simulink model "TVC6DOF_sim"  (R2020b)
settings: Solver=VariableStepAuto  StartTime=0.0  StopTime=7  RelTol=1e-3
values from neighbouring files (symbols this model uses):
  dt = 0.01    [TVC6DOF.m]
  g = 9.81    [TVC6DOF.m]
  Ix_mc = Ix_n+randn*Ix_v    [TVC6DOF.m]
  Ix_n = 0.1    [TVC6DOF.m]
  Iy_mc = Iy_n+randn*Iy_v    [TVC6DOF.m]
  Iy_n = 0.1    [TVC6DOF.m]
  Iz_mc = Iz_n+randn*Iz_v    [TVC6DOF.m]
  Iz_n = 0.1    [TVC6DOF.m]
  kd = 0.1    [TVC6DOF.m]
  ki = 1    [TVC6DOF.m]
  kp = 1    [TVC6DOF.m]
  l_mc = l_n+randn*l_v    [TVC6DOF.m]
  l_n = 0.3    [TVC6DOF.m]
  m_dry_mc = m_dry_n+randn*m_dry_v    [TVC6DOF.m]
  m_dry_n = 0.94    [TVC6DOF.m]
  mis_y_mc = randn*mis_y_v    [TVC6DOF.m]
  mis_z_mc = randn*mis_z_v    [TVC6DOF.m]
  servo_delay_mc = servo_delay_n+randn*servo_delay_v    [TVC6DOF.m]
  static_error_y_mc = randn*static_error_y_v    [TVC6DOF.m]
  static_error_z_mc = randn*static_error_z_v    [TVC6DOF.m]
undefined symbols (not defined in the file or in its folder): sigbuilder_block
settings Model: Creator=govindchari  LastModifiedBy=govindchari

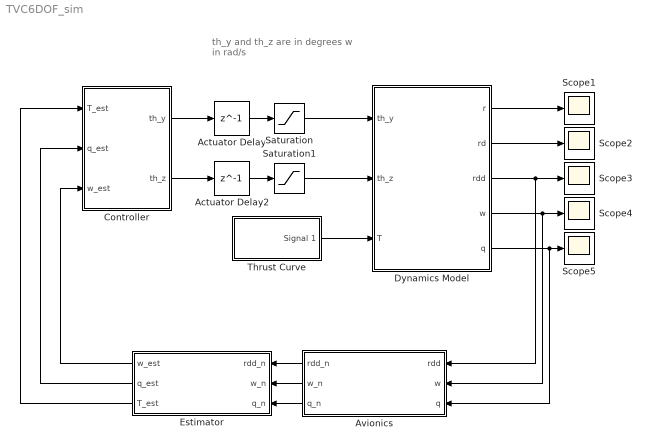
== system TVC6DOF_sim ==
  note: th_y and th_z are in degrees
      |              w in rad/s
  Actuator Delay : Delay  DelayLength=1  InitialCondition=0  SampleTime=servo_delay_mc
  Actuator Delay2 : Delay  DelayLength=1  InitialCondition=0  SampleTime=servo_delay_mc
  Avionics : Subsystem
  Controller : Subsystem
  Dynamics Model : Subsystem
  Estimator : Subsystem
  Saturation : Saturate  UpperLimit=10  LowerLimit=-10
  Saturation1 : Saturate  UpperLimit=10  LowerLimit=-10
  Scope{1..5} (5 alike) : Scope
  Thrust Curve : Subsystem  Tag=STV Subsys  LoadFcn=sigbuilder_block('load');  StartFcn=sigbuilder_block('start');  StopFcn=sigbuilder_block('stop');  ClipboardFcn=sigbuilder_block('clipboard');  mask(Sigbuilder block){tuvar=[0:10]}
      mask help: Simulink:masks:SigbuilderBlock_MD
      mask init:
      | if ~strcmp(get_param(bdroot(gcbh),'SimulationStatus'),'stopped') tuvar = sigbuilder_block('maskInit'); end
      settings: CopyFcn=sigbuilder_block('copy');  DeleteFcn=sigbuilder_block('delete');  ModelCloseFcn=sigbuilder_block('modelClose');  PreSaveFcn=sigbuilder_block('preSave');  PauseFcn=sigbuilder_block('pause');  ContinueFcn=sigbuilder_block('continue');  NameChangeFcn=sigbuilder_block('namechange');  OpenFcn=sigbuilder_block('open',[767 231 550 400 ]);  CloseFcn=sigbuilder_block('close');
      mask Display: plot(0, 0, 100, 100,[2, 2, 32, 32, 2], [68, 8, 8, 68, 68],[32, 2], [38, 38], [32, 19, 2],[53, 60, 44], [32, 17, 17, 2],[16, 16, 31, 31]);txt = getActiveGroup(gcbh);text(2, 100, txt,'verticalAlignment', 'top');
  wires:
  Thrust Curve/1(Signal 1) -> Dynamics Model/3(T)
  Dynamics Model/1(r) -> Scope1/1
  Dynamics Model/2(rd) -> Scope2/1
  Dynamics Model/5(q) -> Avionics/3(q), Scope5/1
  Dynamics Model/4(w) -> Scope4/1, Avionics/2(w)
  Dynamics Model/3(rdd) -> Avionics/1(rdd), Scope3/1
  Avionics/1(rdd_n) -> Estimator/1(rdd_n)
  Avionics/2(w_n) -> Estimator/2(w_n)
  Avionics/3(q_n) -> Estimator/3(q_n)
  Estimator/2(q_est) -> Controller/2(q_est)
  Estimator/3(T_est) -> Controller/1(T_est)
  Controller/2(th_z) -> Actuator Delay2/1
  Actuator Delay2/1 -> Saturation1/1
  Controller/1(th_y) -> Actuator Delay/1
  Actuator Delay/1 -> Saturation/1
  Estimator/1(w_est) -> Controller/3(w_est)
  Saturation/1 -> Dynamics Model/1(th_y)
  Saturation1/1 -> Dynamics Model/2(th_z)

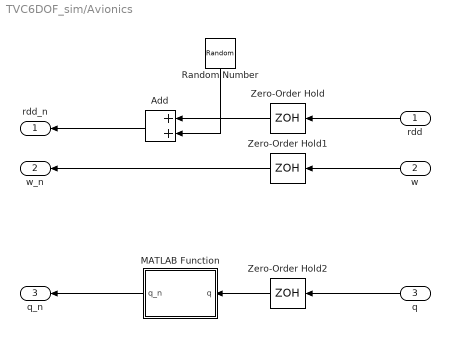
== system TVC6DOF_sim/Avionics ==
  rdd : Inport
  w : Inport  Port=2
  q : Inport  Port=3
  Add : Sum
  MATLAB Function : MATLAB Function  TreatAsAtomicUnit=on
  Random Number : RandomNumber  Mean=0.01  SampleTime=dt
  Zero-Order Hold : ZeroOrderHold  SampleTime=dt
  Zero-Order Hold1 : ZeroOrderHold  SampleTime=dt
  Zero-Order Hold2 : ZeroOrderHold  SampleTime=dt
  rdd_n : Outport
  w_n : Outport  Port=2
  q_n : Outport  Port=3
  wires:
  q/1 -> Zero-Order Hold2/1
  Zero-Order Hold2/1 -> MATLAB Function/1(q)
  w/1 -> Zero-Order Hold1/1
  rdd/1 -> Zero-Order Hold/1
  Zero-Order Hold1/1 -> w_n/1
  Zero-Order Hold/1 -> Add/1
  Add/1 -> rdd_n/1
  Random Number/1 -> Add/2
  MATLAB Function/1(q_n) -> q_n/1

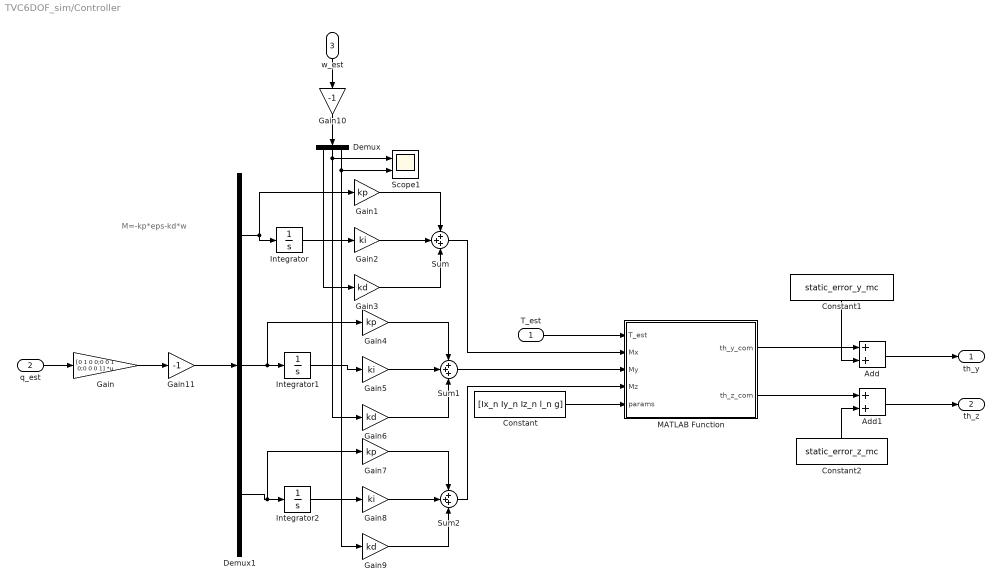
== system TVC6DOF_sim/Controller ==
  note: M=-kp*eps-kd*w
  T_est : Inport
  q_est : Inport  Port=2
  w_est : Inport  Port=3
  Add : Sum
  Add1 : Sum
  Constant : Constant  Value=[Ix_n Iy_n Iz_n l_n g]
  Constant1 : Constant  Value=static_error_y_mc
  Constant2 : Constant  Value=static_error_z_mc
  Demux : Demux  Outputs=3
  Demux1 : Demux  Outputs=3
  Gain : Gain  Gain=[0 1 0 0;0 0 1 0;0 0 0 1]  Multiplication=Matrix(K*u) (u vector)
  Gain1 : Gain  Gain=kp
  Gain10 : Gain  Gain=-1
  Gain11 : Gain  Gain=-1
  Gain2 : Gain  Gain=ki
  Gain3 : Gain  Gain=kd
  Gain4 : Gain  Gain=kp
  Gain5 : Gain  Gain=ki
  Gain6 : Gain  Gain=kd
  Gain7 : Gain  Gain=kp
  Gain8 : Gain  Gain=ki
  Gain9 : Gain  Gain=kd
  Integrator : Integrator  InitialCondition=[0]
  Integrator1 : Integrator  InitialCondition=[0]
  Integrator2 : Integrator  InitialCondition=[0]
  MATLAB Function : MATLAB Function  TreatAsAtomicUnit=on
  Scope1 : Scope  NumInputPorts=2
  Sum : Sum  Inputs=3
  Sum1 : Sum  Inputs=3
  Sum2 : Sum  Inputs=3
  th_y : Outport
  th_z : Outport  Port=2
  wires:
  Integrator/1 -> Gain2/1
  Gain1/1 -> Sum/1
  Gain2/1 -> Sum/2
  Gain3/1 -> Sum/3
  Sum2/1 -> MATLAB Function/4(Mz)
  Sum1/1 -> MATLAB Function/3(My)
  Sum/1 -> MATLAB Function/2(Mx)
  Constant/1 -> MATLAB Function/5(params)
  T_est/1 -> MATLAB Function/1(T_est)
  Demux1/1 -> Integrator/1, Gain1/1
  Integrator1/1 -> Gain5/1
  Gain4/1 -> Sum1/1
  Gain6/1 -> Sum1/3
  Gain5/1 -> Sum1/2
  Demux1/2 -> Gain4/1, Integrator1/1
  Integrator2/1 -> Gain8/1
  Gain7/1 -> Sum2/1
  Gain9/1 -> Sum2/3
  Gain8/1 -> Sum2/2
  Demux1/3 -> Gain7/1, Integrator2/1
  Demux/2 -> Gain6/1, Scope1/1
  Demux/1 -> Gain3/1
  w_est/1 -> Gain10/1
  Gain10/1 -> Demux/1
  q_est/1 -> Gain/1
  Gain/1 -> Gain11/1
  Gain11/1 -> Demux1/1
  Demux/3 -> Scope1/2, Gain9/1
  MATLAB Function/1(th_y_com) -> Add/1
  Add/1 -> th_y/1
  MATLAB Function/2(th_z_com) -> Add1/1
  Add1/1 -> th_z/1
  Constant1/1 -> Add/2
  Constant2/1 -> Add1/2

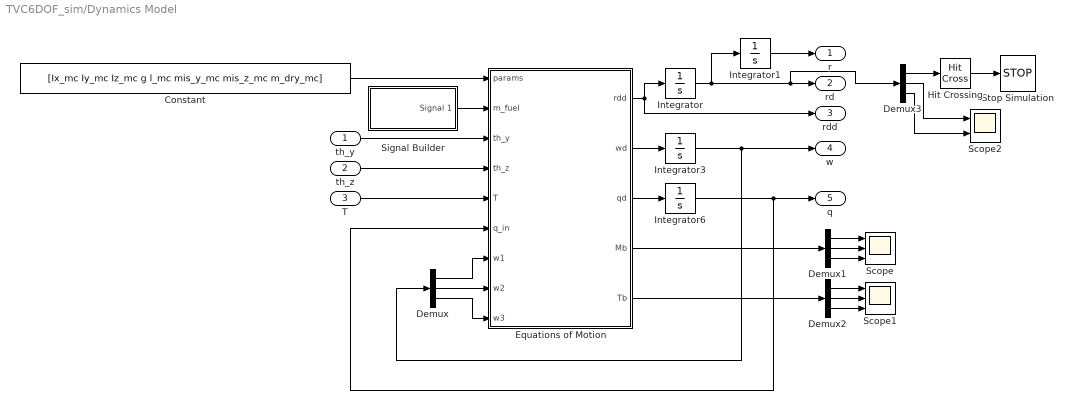
== system TVC6DOF_sim/Dynamics Model ==
  th_y : Inport
  th_z : Inport  Port=2
  T : Inport  Port=3
  Constant : Constant  Value=[Ix_mc Iy_mc Iz_mc g l_mc mis_y_mc mis_z_mc m_dry_mc]
  Demux{,1..3} (4 alike) : Demux  Outputs=3
  Equations of Motion : MATLAB Function  TreatAsAtomicUnit=on
  Hit Crossing : HitCross  HitCrossingOffset=0.01  HitCrossingDirection=falling
  Integrator : Integrator  InitialCondition=[0 0 0]
  Integrator1 : Integrator  InitialCondition=[0 0 0]
  Integrator3 : Integrator  InitialCondition=[0 0 0]
  Integrator6 : Integrator  InitialCondition=[1 0 0 0]
  Scope : Scope  NumInputPorts=3
  Scope1 : Scope  NumInputPorts=3
  Scope2 : Scope  NumInputPorts=2
  Signal Builder : Subsystem  Tag=STV Subsys  LoadFcn=sigbuilder_block('load');  StartFcn=sigbuilder_block('start');  StopFcn=sigbuilder_block('stop');  ClipboardFcn=sigbuilder_block('clipboard');  mask(Sigbuilder block){tuvar=[0:10]}
      mask help: Simulink:masks:SigbuilderBlock_MD
      mask init:
      | if ~strcmp(get_param(bdroot(gcbh),'SimulationStatus'),'stopped') tuvar = sigbuilder_block('maskInit'); end
      settings: CopyFcn=sigbuilder_block('copy');  DeleteFcn=sigbuilder_block('delete');  ModelCloseFcn=sigbuilder_block('modelClose');  PreSaveFcn=sigbuilder_block('preSave');  PauseFcn=sigbuilder_block('pause');  ContinueFcn=sigbuilder_block('continue');  NameChangeFcn=sigbuilder_block('namechange');  OpenFcn=sigbuilder_block('open',[226 376 550 400 ]);  CloseFcn=sigbuilder_block('close');
      mask Display: plot(0, 0, 100, 100,[2, 2, 32, 32, 2], [68, 8, 8, 68, 68],[32, 2], [38, 38], [32, 19, 2],[53, 60, 44], [32, 17, 17, 2],[16, 16, 31, 31]);txt = getActiveGroup(gcbh);text(2, 100, txt,'verticalAlignment', 'top');
  Stop Simulation : Stop
  r : Outport
  rd : Outport  Port=2
  rdd : Outport  Port=3
  w : Outport  Port=4
  q : Outport  Port=5
  wires:
  Constant/1 -> Equations of Motion/1(params)
  th_y/1 -> Equations of Motion/3(th_y)
  th_z/1 -> Equations of Motion/4(th_z)
  Equations of Motion/3(qd) -> Integrator6/1
  Equations of Motion/2(wd) -> Integrator3/1
  Equations of Motion/1(rdd) -> Integrator/1, rdd/1
  T/1 -> Equations of Motion/5(T)
  Integrator/1 -> Integrator1/1, Demux3/1, rd/1
  Integrator1/1 -> r/1
  Demux/1 -> Equations of Motion/7(w1)
  Demux/2 -> Equations of Motion/8(w2)
  Demux/3 -> Equations of Motion/9(w3)
  Integrator6/1 -> Equations of Motion/6(q_in), q/1
  Integrator3/1 -> Demux/1, w/1
  Equations of Motion/4(Mb) -> Demux1/1
  Equations of Motion/5(Tb) -> Demux2/1
  Demux1/1 -> Scope/1
  Demux1/2 -> Scope/2
  Demux1/3 -> Scope/3
  Demux2/1 -> Scope1/1
  Demux2/2 -> Scope1/2
  Demux2/3 -> Scope1/3
  Signal Builder/1(Signal 1) -> Equations of Motion/2(m_fuel)
  Demux3/1 -> Hit Crossing/1
  Hit Crossing/1 -> Stop Simulation/1
  Demux3/2 -> Scope2/1
  Demux3/3 -> Scope2/2

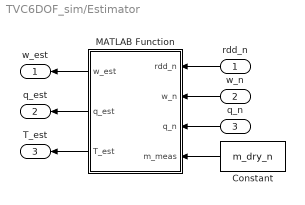
== system TVC6DOF_sim/Estimator ==
  rdd_n : Inport
  w_n : Inport  Port=2
  q_n : Inport  Port=3
  Constant : Constant  Value=m_dry_n
  MATLAB Function : MATLAB Function  TreatAsAtomicUnit=on
  w_est : Outport
  q_est : Outport  Port=2
  T_est : Outport  Port=3
  wires:
  w_n/1 -> MATLAB Function/2(w_n)
  rdd_n/1 -> MATLAB Function/1(rdd_n)
  q_n/1 -> MATLAB Function/3(q_n)
  Constant/1 -> MATLAB Function/4(m_meas)
  MATLAB Function/2(q_est) -> q_est/1
  MATLAB Function/3(T_est) -> T_est/1
  MATLAB Function/1(w_est) -> w_est/1

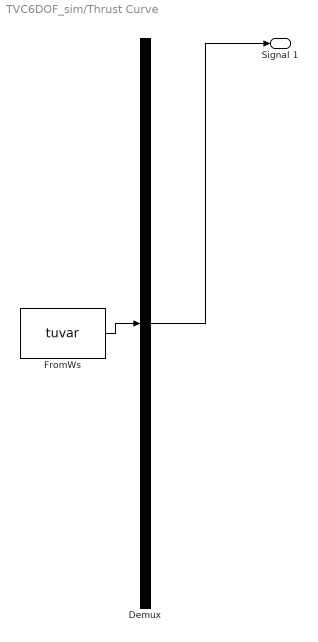
== system TVC6DOF_sim/Thrust Curve ==
  Demux : Demux  Tag=STV Demux  Outputs=1
      settings: DisplayOption=none
  FromWs : FromWorkspace  Tag=STV FromWs  VariableName=tuvar
      SigBuilderData=|
      | common.afterFinalStr = 'Extrapolate'
      | common.sampleTime = 0
      | dataSet.timeRange = [0 10]
      | dataSet.name = 'Group 1'
      | sbobj.Groups.Name = 'Group 1'
      | sbobj.Groups.Signals.Name = 'Signal 1'
      | sbobj.Groups.Signals.XData = [0 0.148 0.228 0.294 0.353 0.382 0.419 0.477 0.52 0.593 0.688 0.855 1.037 1.205 1.423 1.452 1.503 1.736 1.955 2.21 2.494 2.763 3.12 3.382 3.404 3.418 3.45 10]
      | sbobj.Groups.Signals.YData = [0 7.638 12.253 16.391 20.21 22.756 25.26 23.074 20.845 19.093 17.5 16.225 15.427 14.948 14.627 15.741 14.785 14.623 14.303 14.141 13.819 13.338 13.334 13.013 9.352 4.895 0 0]
  Signal 1 : Outport  Tag=STV Outport
  wires:
  Demux/1 -> Signal 1/1
  FromWs/1 -> Demux/1

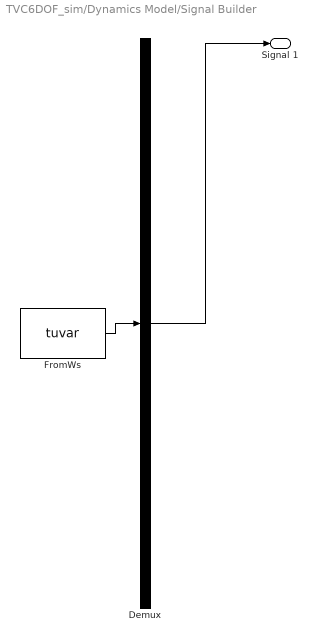
== system TVC6DOF_sim/Dynamics Model/Signal Builder ==
  Demux : Demux  Tag=STV Demux  Outputs=1
      settings: DisplayOption=none
  FromWs : FromWorkspace  Tag=STV FromWs  VariableName=tuvar
      SigBuilderData=|
      | common.afterFinalStr = 'Extrapolate'
      | common.sampleTime = 0
      | dataSet.timeRange = [0 10]
      | dataSet.name = 'Group 1'
      | sbobj.Groups.Name = 'Group 1'
      | sbobj.Groups.Signals.Name = 'Signal 1'
      | sbobj.Groups.Signals.XData = [0 0.148 0.228 0.294 0.419 0.477 0.52 0.593 0.688 0.855 1.037 1.205 1.423 1.452 1.503 1.736 1.955 2.21 2.494 2.763 3.12 3.382 3.404 3.418 3.45 9.8 10]
      | sbobj.Groups.Signals.YData = [60 59.3164 58.3541 57.2108 54.0771 52.3818 51.2397 49.4767 47.3744 43.9685 40.4849 37.3989 33.5 32.9674 32.026 27.8823 24.0514 19.6652 14.8632 10.4455 4.68731 0.51289 0.215344 0.0947253 0 0 0]
  Signal 1 : Outport  Tag=STV Outport
  wires:
  Demux/1 -> Signal 1/1
  FromWs/1 -> Demux/1

== matlab function TVC6DOF_sim/Estimator/MATLAB Function ==
  data: w_est output; rdd_n input; q_est output; T_est output; w_n input; q_n input; m_meas input
function [w_est,q_est,T_est] = estimator(rdd_n,w_n,q_n,m_meas)
    w_est=w_n;
    T_est=norm(rdd_n)*m_meas;
    q_est=q_n;
end

== matlab function TVC6DOF_sim/Dynamics Model/Equations of Motion ==
  data: params input; m_fuel input; th_y input; rdd output; th_z input; T input; q_in input; wd output; qd output; w1 input; w2 input; w3 input; Mb output; Tb output
function [rdd,wd,qd,Mb,Tb] = EOM(params,m_fuel,th_y,th_z,T,q_in,w1,w2,w3)
Ix=params(1);
Iy=params(2);
Iz=params(3);
g=params(4);
l=params(5);
mis_y=params(6);
mis_z=params(7);
m_dry=params(8);
m=m_dry+m_fuel/1000;
wx=w1;
wy=w2;
wz=w3;

if size(q_in)==1
    q_in=[1;0;0;0];
    th_y=0;
    th_z=0;
end
gCb=[cosd(th_z) sind(th_z) 0;-sind(th_z) cosd(th_z) 0;0 0 1]*[cosd(th_y) 0 -sind(th_y);0 1 0;sind(th_y) 0 cosd(th_y)];
Tb=gCb.'*[T;0;0];

r=[-l;mis_y;mis_z];
Mb=cross(r,Tb);
Ti=hamilton(hamilton(q_in,[0;Tb]),conjugate(q_in));

xdd=Ti(2)/m-g;
ydd=Ti(3)/m;
zdd=Ti(4)/m;

rdd=[xdd;ydd;zdd];

wxd=(1/Ix)*(Mb(1)+(Iy-Iz)*wy*wz);
wyd=(1/Iy)*(Mb(2)+(Iz-Ix)*wx*wz);
wzd=(1/Iz)*(Mb(3)+(Ix-Iy)*wx*wy);

wd=[wxd;wyd;wzd];

qd=0.5*hamilton(q_in,[0;wx;wy;wz]);
    function product=hamilton(q,r)
        product=[r(1)*q(1)-r(2)*q(2)-r(3)*q(3)-r(4)*q(4);
                 r(1)*q(2)+r(2)*q(1)-r(3)*q(4)+r(4)*q(3);
                 r(1)*q(3)+r(2)*q(4)+r(3)*q(1)-r(4)*q(2);
                 r(1)*q(4)-r(2)*q(3)+r(3)*q(2)+r(4)*q(1)];
    end

    function q_star=conjugate(q)
        q_star=[q(1);-q(2);-q(3);-q(4)];
    end
end

== matlab function TVC6DOF_sim/Controller/MATLAB Function ==
  data: T_est input; Mx input; th_y_com output; My input; Mz input; params input; th_z_com output
function [th_y_com,th_z_com] = Moments2Commands(T_est,Mx,My,Mz,params)
    Ix=params(1);
    Iy=params(2);
    Iz=params(3);
    l=params(4);
    g=params(5);
    
    Tb=[0;Mz/l;-My/l];  %First component is unknown (free parameter)
    th_y_com=asin(Tb(3)/T_est)*(180/pi);
    th_z_com=asin(Tb(2)/(-T_est*cos((pi*th_y_com)/180)))*(180/pi);   
end

== matlab function TVC6DOF_sim/Avionics/MATLAB Function ==
  data: q input; q_n output
function q_n = quat_corrupt(q)
    angle_var=0.01;
    axis=randn(3,1);
    axis=axis/norm(axis);
    angle=randn*angle_var;
    q_rot=[cos(angle/2);axis(1)*sin(angle/2);axis(2)*sin(angle/2);axis(3)*sin(angle/2)];
    q_n=hamilton(q,q_rot);
    
    function product=hamilton(q,r)
    product=[r(1)*q(1)-r(2)*q(2)-r(3)*q(3)-r(4)*q(4);
             r(1)*q(2)+r(2)*q(1)-r(3)*q(4)+r(4)*q(3);
             r(1)*q(3)+r(2)*q(4)+r(3)*q(1)-r(4)*q(2);
             r(1)*q(4)-r(2)*q(3)+r(3)*q(2)+r(4)*q(1)];
    end
end
